simulink model "ergasia2"  (R2019a)
settings: Solver=VariableStepAuto  StartTime=0.0  StopTime=1  RelTol=1e-3
libraries: commofdm x2, commdigbbndam3 x2, commchan3 x1, commrandsrc3 x1, commsink2 x1
settings Model: Creator=icsd18107  LastModifiedBy=icsd18107
settings DebuggingCC: SFMachineParentedDataDiag=error

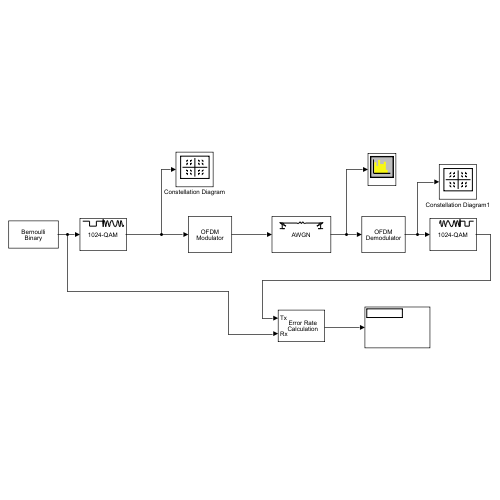
[thumbnail: Simulink's stored preview of the top-level diagram]
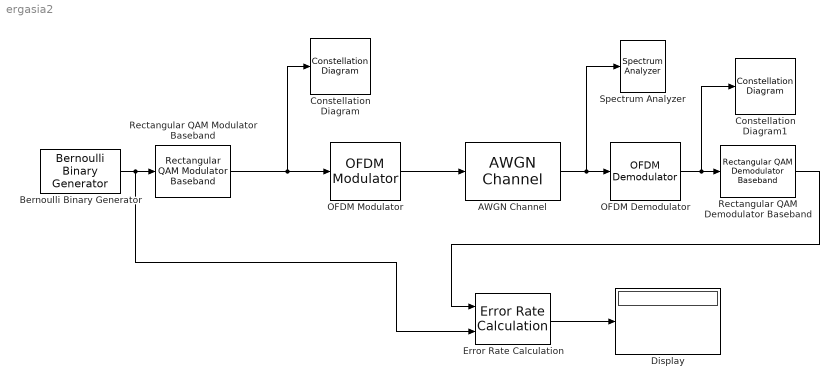
== system ergasia2 ==
  AWGN Channel : commchan3/AWGN Channel  InputProcessing=Columns as channels (frame based)  seed=67  noiseMode="Signal to noise ratio  (SNR)"  EbNodB=10  EsNodB=10  SNRdB=15  bitsPerSym=1  Ps=1  Tsym=1  variance=1
  Bernoulli Binary Generator : commrandsrc3/Bernoulli Binary Generator  ProbabilityOfZero=0.55  SeedSource=Parameter  Seed=20394875  SampleTime=1/600*1e-3  SamplesPerFrame=600  OutputDataType=boolean  SimulateUsing=Interpreted execution
  Constellation Diagram : ConstellationDiagram
  Constellation Diagram1 : ConstellationDiagram
  Display : Display
  Error Rate Calculation : commsink2/Error Rate Calculation  N=0  st_delay=0  cp_mode=Entire frame  subframe=[]  PMode=Port  WsName=ErrorVec  RsMode2=off  stop=off  numErr=100  maxBits=1e6
  OFDM Demodulator : commofdm/OFDM Demodulator  StatePerturbationForJacobian=1.0e-05  FFTLength=87  NumGuardBandCarriers=[20; 6]  RemoveDCCarrier=on  PilotOutputPort=off  PilotCarrierIndices=[12; 26; 40; 54]  CyclicPrefixLength=16  NumSymbols=1  NumReceiveAntennas=1  SimulateUsing=Interpreted execution
      settings: SourceProductBaseCode=CM
  OFDM Modulator : commofdm/OFDM Modulator  StatePerturbationForJacobian=1.0e-05  FFTLength=87  NumGuardBandCarriers=[20; 6]  InsertDCNull=on  PilotInputPort=off  PilotCarrierIndices=[12; 26; 40; 54]  CyclicPrefixLength=16  Windowing=on  WindowLength=1  NumSymbols=1  NumTransmitAntennas=1  SimulateUsing=Interpreted execution
      settings: SourceProductBaseCode=CM
  Rectangular QAM Demodulator Baseband : commdigbbndam3/Rectangular QAM Demodulator Baseband  M=1024  OutType=Bit  DecType=Hard decision  VarSource=Dialog  Variance=1  Dec=Gray  Mapping=[0:15]  PowType=Min. distance between symbols  MinDist=2  AvgPow=1  PeakPow=1  Ph=0  outDtype1=boolean  outDtype2=Inherit via internal rule  derotateFactorWordLen=16  derotateFactorDataTypeStr=Inherit: Same word length as input  derotateFactorLastDataTypeStr=Inherit: Same word length as input  denormFactorWordLen=16  denormFactorDataTypeStr=Inherit: Same word length as input  denormFactorLastDataTypeStr=Inherit: Same word length as input  prodOutWordLen=32  prodOutOverflowMode=Wrap  prodOutRoundingMode=Floor  prodOutOvFlMode=off  prodOutOvFlModeLastStrValue=off  sumWordLen=32
  Rectangular QAM Modulator Baseband : commdigbbndam3/Rectangular QAM Modulator Baseband  M=1024  InType=Bit  Enc=Gray  Mapping=[0:15]  PowType=Min. distance between symbols  MinDist=2  AvgPow=1  PeakPow=1  Ph=0  outDtype=double  outWordLen=16  outUDDataType=sfix(16)  outFracLenMode=Best precision  outFracLen=15  outDataTypeStr=double  outLastDataTypeStr=double
  Spectrum Analyzer : SpectrumAnalyzer
  wires:
  Bernoulli Binary Generator/1 -> Error Rate Calculation/2, Rectangular QAM Modulator Baseband/1
  OFDM Modulator/1 -> AWGN Channel/1
  AWGN Channel/1 -> Spectrum Analyzer/1, OFDM Demodulator/1
  OFDM Demodulator/1 -> Constellation Diagram1/1, Rectangular QAM Demodulator Baseband/1
  Error Rate Calculation/1 -> Display/1
  Rectangular QAM Demodulator Baseband/1 -> Error Rate Calculation/1
  Rectangular QAM Modulator Baseband/1 -> OFDM Modulator/1, Constellation Diagram/1
